simulink model "Dual_Clutch_Trans_SDO_ORIG"  (R2015b)
settings: Solver=ode1  StartTime=0.0  StopTime=15  MaxStep=0.1  RelTol=1e-3
PreLoadFcn:
  | load UrbanCycle1;
  | load UrbanCycle2;
  | load UrbanCycle3;
  | load UrbanCycle4;
  | load UrbanCycle5;
  | load UrbanCycle6;
  | load UrbanCycle7;
  | load UrbanCycle8;
  | Shift_Gear_Delay = 50;
  | Ratio_Time_Const = 0.1;
  | Drive_Cycle_Num = 7;
  | load RefRPMData;
PostLoadFcn:
  | warning off Simulink:SampleTime:TsPropEnabOutputsChangeNotAligned;
  | warning off Simulink:blocks:MatchingFromNotFound
  | warning off Simulink:blocks:MatchingGotoNotFound
  | warning off Simulink:Engine:OutputNotConnected
  | warning off Simulink:Engine:LineWithoutDst
  | warning off Simulink:Engine:UINotUpdatedDuringRapidAccelSim
  | warning off Simulink:Commands:SetParamLinkChangeWarn
  | warning off Simulink:Engine:SaveWithParameterizedLinks_Warning
undefined symbols (not defined in the file or in its folder): DCT_Param, Downshift_Speeds, sigbuilder_block, Upshift_Speeds
libraries: fl_lib x8, nesl_utility x7, sdl_lib x3, simulink x3, DCT_Vehicle_Dynamics_Lib x1
(part 1 of 2)
Description:
  | Vehicle With Dual Clutch Transmission
  | 
  | The vehicle simulated in this demo has a five-speed automatic dual-clutch
  | transmission. The transmission controller converts the pedal deflection
  | into a demanded torque. This demanded torque is then passed to the
  | engine management. The pedal deflection and the vehicle speed are also
  | used by the transmission controller to determine when the gear shifts
  | should occur. Gear shifts are implemented via the two clutches, one clutch
  | pressure being ramped up as the other clutch pressure is ramped down.
  | Gear pre-selection is used to ensure that the correct gear is fully selected
  | before the on-going clutch is enabled. Double-click on the two blocks
  | labeled "Configure for ...." to switch between variable and fixed-step solvers.
  | 
  | 
  | Copyright 2008-2016 The MathWorks, Inc.
settings Model: ParamWorkspaceSource=ReferencedWorkspace  ExtModeTrigDuration=200  ExtModeLogAll=off  TunableVars=Downshift_Speeds,Pedal_Positions,Upshift_Speeds  TunableVarsStorageClass=Auto,Auto,Auto  TunableVarsTypeQualifier=,,  Creator=MathWorks  LastModifiedBy=smiller
settings SolverCC: MaxConsecutiveZCs=10  MaxConsecutiveMinStep=5  EnableConcurrentExecution=on  AutoInsertRateTranBlk=on
settings DataIOCC: MaxDataPoints=1  SaveFormat=StructureWithTime  SaveOutput=off  DSMLogging=off  SaveTime=off  SignalLoggingName=SDO_logsout
settings OptimizationCC: BlockReduction=off  DefaultParameterBehavior=Inlined  OptimizeBlockIOStorage=off  BufferReuse=off  GlobalBufferReuse=off  ExpressionFolding=off  ExpressionDepthLimit=2147483647  LocalBlockOutputs=off
settings DebuggingCC: AlgebraicLoopMsg=error  UnderspecifiedInitializationDetection=Classic  MergeDetectMultiDrivingBlocksExec=none  IgnoredZcDiagnostic=none  MultiTaskRateTransMsg=warning  FcnCallInpInsideContextMsg=UseLocalSettings  StateNameClashWarn=warning
settings HardwareCC: ProdBitPerPointer=32  ProdLargestAtomicFloat=None  ProdWordSize=32  ProdLongLongMode=on  ProdHWDeviceType=Generic->32-bit x86 compatible
settings RTWCC: SystemTargetFile=slrt.tlc  TemplateMakefile=slrt_default_tmf  Description=Simulink Real-Time  RTWCompilerOptimization=on
settings ConfigComp: CovModelRefEnable=Off
settings SimscapeCC: ExplicitSolverDiagnosticOptions=none  SimscapeLogLimitData=off  SimscapeLogDataHistory=50000

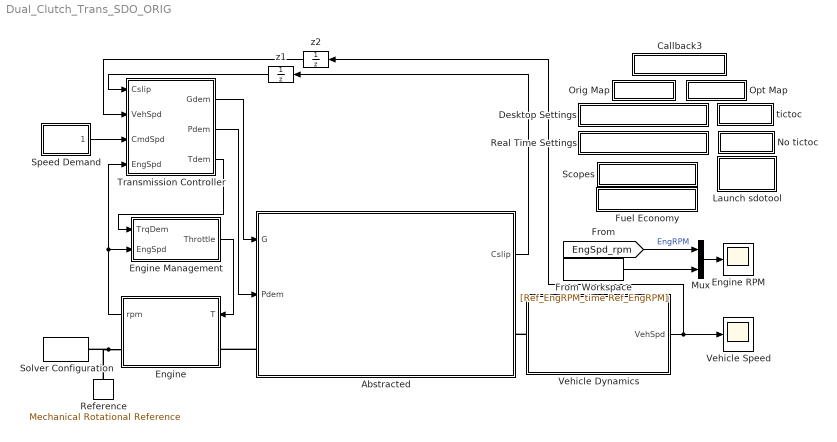
== system Dual_Clutch_Trans_SDO_ORIG ==
  Abstracted : Subsystem
      mask Display:
      | image(imread('DCT_Transmission_Abstracted_IMAGE2.jpg'));
      | port_label('input',1,'G')
      | port_label('input',2,'Pdem')
      | port_label('output',1,'Cslip')
      | color('red');
      | port_label('LConn',1,'B')
      | port_label('RConn',1,'F')
  Callback3 : Subsystem
      settings: OpenFcn=Plot_Gear_Shift_Schedule(Pedal_Positions,Upshift_Speeds, Downshift_Speeds);
      mask Display: disp('Shift Schedule')
  Desktop Settings : Subsystem
      settings: OpenFcn=|
      | set_param(gcs,'solver','ode23t')
      | set_param(sprintf([gcs '/Solver\nConfiguration']),'UseLocalSolver','off')
      | 
      | set_param(sprintf([gcs '/Solver\nConfiguration']),'DoFixedCost','off')
      mask Display: disp('Desktop Settings')
  Engine : Subsystem
      mask Display:
      | plot([200.294537656123;201.704177092068;202.879954177142;203.81054553527;204.486989062962;204.902770239264;205.053884864158;204.938877621199;204.558856093007;203.917480094638;203.02092642757;201.877829393721;200.499197642409;198.898308151034;197.090578360535;195.093417696999;192.926059909376;191.349221415216], [79.0962651705123;81.4129472419303;83.856642682368;86.4038173688741;89.0299406167901;91.7097214236537;94.4173520353776;97.1267564890293;99.8118417386092;102.446748945347;105.006102512455;107.465254465996;109.80052182835;111.989414698229;114.010852840726;115.845368701499;117.475294889959;118.468271604945])
      | plot([180.070315486255;177.215173525063;174.340173090774;171.473002009205;168.641272705228;165.872256280019;163.192619875453;160.628169854943;158.203603274058;155.942270034374;153.865948011161;151.994633320535;150.346347745932;148.936965178479;147.780058742747;146.886770080143;146.265702048809;145.922835873396;145.861473542603;146.08220600922;146.58290749893;147.358755982674;148.402279615432;149.703428694174;151.249672441989;153.026119686324;155.015662269112;157.199139807684;159.555524219735;162.062122235246;164.694793945081;167.42818528151;170.23597219174;173.091114152932;175.966114587221;178.83328566879;181.665014972767;184.434031397976;185.486929355725], [123.25590763568;123.598773811093;123.660136141886;123.439403675268;122.938702185559;122.162853701815;121.119330069056;119.818180990315;118.2719372425;116.495489998164;114.505947415377;112.322469876805;109.966085464754;107.459487449243;104.826815739408;102.093424402979;99.2856374927491;96.4304955315569;93.5554950972677;90.688324015699;87.8565947117214;85.0875782865128;82.4079418819464;79.8434918614364;77.4189252805513;75.1575920408679;73.081270017655;71.2099553270291;69.5616697524256;68.1522871849724;66.9953807492411;66.1020920866371;65.4810240553025;65.1381578798894;65.0767955490969;65.2975280157144;65.7982295054238;66.5740779891678;66.9481130562871])
      | plot([182.088349247351;182.056804583223;181.962474383197;181.806267098667;181.589687091173;181.314820144583;180.98431337785;180.601349751811;180.169617415534;179.693274187426;179.176907513169;178.625490286111;178.044332955585;177.439032384376;176.815417947876;176.17949539401;175.537389004603;174.895282615196;174.25936006133;173.63574562483;173.030445053621;172.449287723095;171.897870496037;171.38150382178;170.905160593672;170.473428257395;170.090464631356;169.759957864623;169.485090918033;169.268510910539;169.112303626009;169.017973425983;168.986428761855;169.017973425983;169.112303626009;169.268510910539;169.485090918033;169.759957864623;170.090464631356;170.473428257395;170.905160593672;171.38150382178;171.897870496037;172.449287723095;173.030445053621;173.63574562483;174.25936006133;174.895282615196;175.537389004603;176.17949539401;176.815417947876;177.439032384376;178.044332955585;178.625490286111;179.176907513169;179.693274187426;180.169617415534;180.601349751811;180.98431337785;181.314820144583;181.589687091173;181.806267098667;181.962474383197;182.056804583223;182.088349247351;182.088349247351], [94.3432759959251;93.7073437064164;93.0775357924916;92.4599176486499;91.8604372752408;91.2848679959696;90.7387528576339;90.2273512475527;89.7555882427917;89.3280071789786;88.9487258954975;88.6213970784445;88.3491730832641;88.1346755758426;87.9799702844327;87.8865471055612;87.8553057555109;87.8865471055612;87.9799702844327;88.1346755758426;88.3491730832641;88.6213970784445;88.9487258954975;89.3280071789786;89.7555882427917;90.2273512475527;90.7387528576339;91.2848679959696;91.8604372752408;92.4599176486499;93.0775357924916;93.7073437064164;94.3432759959251;94.9792082854337;95.6090161993586;96.2266343432003;96.8261147166093;97.4016839958805;97.9477991342162;98.4592007442974;98.9309637490584;99.3585448128716;99.7378260963527;100.065154913406;100.337378908586;100.551876416008;100.706581707417;100.800004886289;100.831246236339;100.800004886289;100.706581707417;100.551876416008;100.337378908586;100.065154913406;99.7378260963526;99.3585448128716;98.9309637490584;98.4592007442974;97.9477991342162;97.4016839958805;96.8261147166093;96.2266343432003;95.6090161993586;94.9792082854338;94.3432759959251;94.3432759959251])
      | plot([201.615249970928;201.583705306799;201.489375106774;201.333167822243;201.11658781475;200.84172086816;200.511214101427;200.128250475388;199.69651813911;199.220174911002;198.703808236745;198.152391009688;197.571233679162;196.965933107953;196.342318671452;195.706396117586;195.06428972818;194.422183338773;193.786260784907;193.162646348407;192.557345777197;191.976188446671;191.424771219614;190.908404545357;190.432061317249;190.000328980971;189.617365354932;189.286858588199;189.011991641609;188.795411634116;188.639204349585;188.54487414956;188.513329485431;188.54487414956;188.639204349585;188.795411634116;189.011991641609;189.286858588199;189.617365354932;190.000328980971;190.432061317249;190.908404545357;191.424771219614;191.976188446671;192.557345777197;193.162646348407;193.786260784907;194.422183338773;195.06428972818;195.706396117586;196.342318671452;196.965933107953;197.571233679162;198.152391009688;198.703808236745;199.220174911002;199.69651813911;200.128250475388;200.511214101427;200.84172086816;201.11658781475;201.333167822243;201.489375106774;201.583705306799;201.615249970928;201.615249970928], [74.7533852700144;74.1174529805057;73.487645066581;72.8700269227392;72.2705465493302;71.694977270059;71.1488621317233;70.6374605216421;70.165697516881;69.7381164530679;69.3588351695868;69.0315063525339;68.7592823573535;68.5447848499319;68.390079558522;68.2966563796505;68.2654150296003;68.2966563796505;68.390079558522;68.5447848499319;68.7592823573535;69.0315063525339;69.3588351695868;69.7381164530679;70.165697516881;70.6374605216421;71.1488621317233;71.694977270059;72.2705465493302;72.8700269227392;73.487645066581;74.1174529805057;74.7533852700144;75.3893175595231;76.0191254734479;76.6367436172896;77.2362239906986;77.8117932699698;78.3579084083055;78.8693100183867;79.3410730231478;79.7686540869609;80.147935370442;80.4752641874949;80.7474881826754;80.9619856900969;81.1166909815068;81.2101141603783;81.2413555104285;81.2101141603783;81.1166909815068;80.9619856900969;80.7474881826753;80.4752641874949;80.147935370442;79.7686540869609;79.3410730231478;78.8693100183867;78.3579084083055;77.8117932699698;77.2362239906986;76.6367436172896;76.0191254734479;75.3893175595231;74.7533852700145;74.7533852700144])
      | plot([201.615249970928;201.583705306799;201.489375106774;201.333167822243;201.11658781475;200.84172086816;200.511214101427;200.128250475388;199.69651813911;199.220174911002;198.703808236745;198.152391009688;197.571233679162;196.965933107953;196.342318671452;195.706396117586;195.06428972818;194.422183338773;193.786260784907;193.162646348407;192.557345777197;191.976188446671;191.424771219614;190.908404545357;190.432061317249;190.000328980971;189.617365354932;189.286858588199;189.011991641609;188.795411634116;188.639204349585;188.54487414956;188.513329485431;188.54487414956;188.639204349585;188.795411634116;189.011991641609;189.286858588199;189.617365354932;190.000328980971;190.432061317249;190.908404545357;191.424771219614;191.976188446671;192.557345777197;193.162646348407;193.786260784907;194.422183338773;195.06428972818;195.706396117586;196.342318671452;196.965933107953;197.571233679162;198.152391009688;198.703808236745;199.220174911002;199.69651813911;200.128250475388;200.511214101427;200.84172086816;201.11658781475;201.333167822243;201.489375106774;201.583705306799;201.615249970928;201.615249970928], [74.7533852700144;74.1174529805057;73.487645066581;72.8700269227392;72.2705465493302;71.694977270059;71.1488621317233;70.6374605216421;70.165697516881;69.7381164530679;69.3588351695868;69.0315063525339;68.7592823573535;68.5447848499319;68.390079558522;68.2966563796505;68.2654150296003;68.2966563796505;68.390079558522;68.5447848499319;68.7592823573535;69.0315063525339;69.3588351695868;69.7381164530679;70.165697516881;70.6374605216421;71.1488621317233;71.694977270059;72.2705465493302;72.8700269227392;73.487645066581;74.1174529805057;74.7533852700144;75.3893175595231;76.0191254734479;76.6367436172896;77.2362239906986;77.8117932699698;78.3579084083055;78.8693100183867;79.3410730231478;79.7686540869609;80.147935370442;80.4752641874949;80.7474881826754;80.9619856900969;81.1166909815068;81.2101141603783;81.2413555104285;81.2101141603783;81.1166909815068;80.9619856900969;80.7474881826753;80.4752641874949;80.147935370442;79.7686540869609;79.3410730231478;78.8693100183867;78.3579084083055;77.8117932699698;77.2362239906986;76.6367436172896;76.0191254734479;75.3893175595231;74.7533852700145;74.7533852700144])
      | plot([142.90856779553;142.90856779553;208.103220211342;208.103220211342], [139.948037685826;218.181620584801;218.181620584801;139.948037685826])
      | plot([142.90856779553;208.103220211342], [179.064829135314;179.064829135314])
      | plot([149.459528038278;149.459528038278], [179.064829135314;172.576858894899])
      | plot([201.615249970928;201.615249970928], [179.064829135314;172.576858894899])
      | plot([142.90856779553;208.103220211342;208.103220211342;142.90856779553;142.90856779553], [179.064829135314;179.064829135314;152.986968168989;152.986968168989;179.064829135314])
      | plot([142.90856779553;208.103220211342], [192.103759618476;192.103759618476])
      | plot([180.639579193667;200.229469919577], [99.0045361686498;79.4776354450732])
      | plot([173.332738922909;192.92262964882], [87.8553057555109;68.3284050319344])
      | plot([183.663099305704;200.481429928914], [153.553878189996;76.9580353517085])
      | plot([184.544959338382;174.970478983596], [95.0361660216004;153.553878189996])
      | plot([183.474129298702;186.749609420076;206.654450157657;201.615249970928;197.961829835549], [76.9580353517085;62.0923948008567;67.8874750155956;88.1702557671815;87.7923157531768])
      | plot([164.199188584462;187.694459455088], [94.7842060122639;95.1621460262686])
      | plot([175.537389004603;175.285428995267], [106.50034644641;81.9342455361038])
      | plot([142.90856779553;208.103220211342], [172.576858894899;172.576858894899])
      | plot([297.86397353746;357.389525743201], [71.0999651346356;71.0999651346356])
      | plot([269.518472487107;297.86397353746;297.86397353746;269.518472487107;269.518472487107], [85.2727156598121;85.2727156598121;56.927214609459;56.927214609459;85.2727156598121])
      | plot([258.180272066966;269.518472487107;269.518472487107;258.180272066966], [42.7544640842825;42.7544640842825;99.4454661849886;99.4454661849886])
      | plot([108.893966535106;108.245686045801;107.603648851995;106.974038122836;106.362917353826;105.776171972045;105.219452656266;104.698120917834;104.217197466378;103.781313857637;103.394667889039;103.060983172626;102.783473274627;102.564810767061;102.40710148941;102.31186426823;102.280016290024;102.280016290024;102.31186426823;102.40710148941;102.564810767061;102.783473274627;103.060983172626;103.394667889039;103.781313857637;104.217197466378;104.698120917834;105.219452656266;105.776171972045;106.362917353826;106.974038122836;107.603648851995;108.245686045801;108.893966535106;249.67662175186;250.324902241165;250.966939434972;251.596550164131;252.20767093314;252.794416314921;253.3511356307;253.872467369133;254.353390820588;254.78927442933;255.175920397927;255.50960511434;255.787115012339;256.005777519905;256.163486797556;256.258724018736;256.290571996942;256.290571996942;256.258724018736;256.163486797556;256.005777519905;255.787115012339;255.50960511434;255.175920397927;254.78927442933;254.353390820588;253.872467369133;253.3511356307;252.794416314921;252.20767093314;251.596550164131;250.966939434972;250.324902241165;249.67662175186;108.893966535106], [233.173241140321;233.141393162114;233.046155940935;232.888446663284;232.669784155718;232.392274257719;232.058589541306;231.671943572708;231.236059963967;230.755136512511;230.233804774079;229.6770854583;229.090340076519;228.479219307509;227.84960857835;227.207571384544;226.559290895239;46.5338642243296;45.8855837350246;45.2435465412178;44.6139358120588;44.0028150430496;43.4160696612682;42.8593503454891;42.3380186070568;41.8570951556014;41.4212115468599;41.0345655782626;40.7008808618494;40.42337096385;40.2047084562844;40.0469991786335;39.9517619574538;39.9199139792472;39.9199139792472;39.9517619574538;40.0469991786335;40.2047084562844;40.42337096385;40.7008808618494;41.0345655782626;41.4212115468599;41.8570951556014;42.3380186070568;42.8593503454891;43.4160696612682;44.0028150430496;44.6139358120588;45.2435465412178;45.8855837350246;46.5338642243296;226.559290895239;227.207571384544;227.84960857835;228.479219307509;229.090340076519;229.6770854583;230.233804774079;230.755136512511;231.236059963967;231.671943572708;232.058589541306;232.392274257719;232.669784155718;232.888446663284;233.046155940935;233.141393162114;233.173241140321;233.173241140321])
      | patch([0;354.791188146919;354.791188146919;0;0;0.472425017505884;0.472425017505884;354.318763129413;354.318763129413;0.472425017505884;0], [283.927435521036;283.927435521036;0;0;283.927435521036;283.455010503531;0.472425017505884;0.472425017505884;283.455010503531;283.455010503531;283.927435521036], [1;1;1])
      | plot([102.280016290024;0.236212508752942], [71.0999651346356;71.0999651346356])
      | ;
      | color('black');
      | port_label('input', 1,'T')
      | port_label('output', 1,'rpm')
      | port_label('RConn', 1,'B')
      | port_label('LConn', 1,'F')
  Engine Management : Subsystem
  Engine RPM : Scope
  From Workspace : FromWorkspace  VariableName=[Ref_EngRPM_time Ref_EngRPM]  SampleTime=0.01
  Fuel Economy : Subsystem  mask(Data Acquisition){}
      mask Display: disp('Fuel Economy');
  Launch sdotool : Subsystem
      settings: OpenFcn=|
      | load([bdroot '_sdosession']);
      | sdotool(SDOSessionData);
      mask Display: disp('Launch\nsdotool')
  Mux : Mux  Inputs=2
  No tictoc : Subsystem
      settings: OpenFcn=|
      | set_param(bdroot,'StartFcn','');
      | set_param(bdroot,'StopFcn','');
      mask Display: disp('No tictoc')
  Opt Map : Subsystem
      settings: OpenFcn=|
      | Upshift_Speeds = DCT_Param.Shift_Map_OPT.Upshift_Speeds;
      | Downshift_Speeds = DCT_Param.Shift_Map_OPT.Downshift_Speeds;
      | Pedal_Positions = DCT_Param.Shift_Map_OPT.Pedal_Positions;
      mask Display: disp('Opt Map')
  Orig Map : Subsystem
      settings: OpenFcn=|
      | Upshift_Speeds = DCT_Param.Shift_Map_ORIG.Upshift_Speeds;
      | Downshift_Speeds = DCT_Param.Shift_Map_ORIG.Downshift_Speeds;
      | Pedal_Positions = DCT_Param.Shift_Map_ORIG.Pedal_Positions;
      mask Display: disp('Orig Map')
  Real Time Settings : Subsystem
      settings: OpenFcn=|
      | set_param(gcs,'solver','ode1')
      | set_param(sprintf([gcs '/Solver\nConfiguration']),'UseLocalSolver','on')
      | 
      | set_param(sprintf([gcs '/Solver\nConfiguration']),'DoFixedCost','on')
      mask Display: disp('Real Time Settings')
  Reference : fl_lib/Mechanical/Rotational Elements/Mechanical Rotational Reference
  Scopes : Subsystem
      mask Display: disp('Scopes')
  Solver Configuration : nesl_utility/Solver Configuration  PhysicalDomain=network_engine_domain  SubClassName=solver  LeftPortType=input  RightPortType=generic  Accelerate=off  Tones=[]  Harmonics=[]  SimulateNoise=off  Profile=off  UseLocalSampling=off  EnableSwitchedLinearOptims=on  FrequencyDomain=off  UseCCode=off  RelTol=0.001  AbsTol=1e-06  MinStep=1e-09  ToWorkspace=off  RevertToSquareIcSolve=off  NumHomotopyIterations=100  PhasorMode=off  PhasorModeNumHarmonics=1  DoDC=off  ResidualTolerance=1e-9  UseLocalSolver=on  LocalSolverChoice=NE_BACKWARD_EULER_ADVANCER  LocalSolverSampleTime=.005  DoFixedCost=on  MaxNonlinIter=2  MaxModeIter=2  LinearAlgebra=Sparse  DelaysMemoryBudget=1024  AutomaticFiltering=on  FilteringTimeConstant=0.001
  Speed Demand : Subsystem
      mask Display:
      | plotstr=['UrbanCycle' evalin('base','num2str(Drive_Cycle_Num)')];
      | plot(evalin('base',[plotstr '.time']),evalin('base',[plotstr '.SpdKph']));
      | text(evalin('base',['0.7*max(' plotstr '.time)']),evalin('base',['0.25*max(' plotstr '.SpdKph)']),evalin('base','num2str(Drive_Cycle_Num)'));
  Transmission Controller : Subsystem
  Vehicle Dynamics : Subsystem  BlockChoice=Simple
      settings: AttributesFormatString=%<BlockChoice>  TemplateBlock=DCT_Vehicle_Dynamics_Lib/Vehicle Dynamics  MemberBlocks=Full,Simple
      mask Display:
      | port_label('LConn',1,'Sh');
      | port_label('output',1,'Spd');
  Vehicle Speed : Scope
  tictoc : Subsystem
      settings: OpenFcn=|
      | set_param(bdroot,'StartFcn','tic;');
      | set_param(bdroot,'StopFcn','Elapsed_Sim_Time = toc; disp([''Elapsed time for '' bdroot '' = '' num2str(Elapsed_Sim_Time)])');
      mask Display: disp('tictoc')
  z1 : UnitDelay  SampleTime=0.01
  z2 : UnitDelay  SampleTime=0.01
  wires:
  Transmission Controller/2(Pdem) -> Abstracted/2(Pdem)
  Transmission Controller/1(Gdem) -> Abstracted/1(G)
  z1/1 -> Transmission Controller/1(Cslip)
  Engine Management/1(Throttle) -> Engine/1(T)
  Transmission Controller/3(Tdem) -> Engine Management/1(TrqDem)
  Engine/1(rpm) -> Transmission Controller/4(EngSpd), Engine Management/2(EngSpd)
  Abstracted/1(Cslip) -> z1/1
  Vehicle Dynamics/1(VehSpd) -> Vehicle Speed/1, z2/1
  Speed Demand/1(Speed Command) -> Transmission Controller/3(CmdSpd)
  z2/1 -> Transmission Controller/2(VehSpd)
  [EngSpd_rpm] -> Mux/1  "EngRPM"
  From Workspace/1 -> Mux/2
  Mux/1 -> Engine RPM/1
  connections:
  Engine/RConn1 -- Reference/LConn1 -- Solver Configuration/RConn1
  Abstracted/LConn1 -- Engine/LConn1
  Vehicle Dynamics/LConn1 -- Abstracted/RConn1

== system Dual_Clutch_Trans_SDO_ORIG/Abstracted ==
  G : Inport
  Pdem : Inport  Port=2
  Clutches : Subsystem
      mask Display: image(imread('DCT_Clutches_Abstracted_IMAGE.jpg'));
  Gears : Subsystem
      mask Display: image(imread('DCT_Gears_Abstracted_IMAGE.jpg'));
  Shaft Inertia Output Shaft : fl_lib/Mechanical/Rotational Elements/Inertia  inertia=DCT_Param.Transmission.Shaft_Inertia_Output kg*m^2  w_specify=on  w_priority=High  w=DCT_Param.Transmission.Shaft_Velocity_Output rad/s  t_specify=off  t_priority=None  t=0 N*m
  B : PMIOPort  Port=1  Side=Left
  F : PMIOPort  Port=2  Side=Right
  Cslip : Outport
  wires:
  Pdem/1 -> Clutches/1(Pdem)
  Clutches/1(Cslip) -> Cslip/1
  G/1 -> Gears/1(G)
  connections:
  B/RConn1 -- Clutches/LConn1
  Clutches/RConn1 -- Gears/LConn1
  Gears/RConn1 -- F/RConn1 -- Shaft Inertia Output Shaft/LConn1

== system Dual_Clutch_Trans_SDO_ORIG/Callback3 ==

== system Dual_Clutch_Trans_SDO_ORIG/Desktop Settings ==

== system Dual_Clutch_Trans_SDO_ORIG/Engine ==
  T : Inport
  Generic Engine : sdl_lib/Engines/Generic Engine  model_parameterization=1  engine_type=1  P_max=DCT_Param.ICE.Max_Power W  w_P_max=DCT_Param.ICE.Speed_At_Max_Power rpm  w_max=DCT_Param.ICE.Max_Speed rpm  w_min=DCT_Param.ICE.Stall_Speed rpm  w_tab=[ 500 1000 2e+3 3e+3 4e+3 5e+3 6e+3 7e+3 ] rpm  trq_tab=[ 380 380 380 380 350 280 200 80 ] N*m  pwr_tab=[ 2e+4 4e+4 7.8e+4 1.2e+5 1.45e+5 1.48e+5 1.25e+5 6e+4 ] W  interp_method=1  model_inertia=1  inertia=DCT_Param.ICE.Shaft_Inertia kg*m^2  initial_velocity=DCT_Param.ICE.Initial_Velocity rpm  model_time_constant=1  time_constant=DCT_Param.ICE.Engine_Time_Constant s  T0=DCT_Param.ICE.Initial_Normalized_Throttle  w_thr=DCT_Param.ICE.Speed_Threshold rpm  idle_speed=0  idle_speed_reference=1000 rpm  tau_controller=1 s  idle_w_thr=1 rpm  fc_model=1  fc_per_rev=25 mg/rev  displaced_volume=400 cm^3  rev_per_cycle=2  fc_w_tab=[ 1000 2e+3 3e+3 4e+3 5e+3 6e+3 ] rpm  fc_trq_tab=[ 0 80 160 200 240 320 360 400 ] N*m  fc_tab=[ 0.5 0.9 1.4 1.6 1.9 2.7 3.4 4.4; 1 1.7 2.7 3.1 3.6 5 6 7.4; 1.4 2.7 4 4.8 5.6 7.5 8.5 10.5; 2 3.6 5.8 6.7 8 10.4 11.7 13.3; 2.5 4.8 7.9 9.4 10.8 14 16.2 18.6; 3.1 6 10.3 11.9 13.8 18.4 22 26.5 ] g/s  bmep_tab=[ 0 250 500 625 750 1000 1.15e+3 1.25e+3 ] kPa  bsfc_tab=[ 410 380 300 280 270 290 320 380; 410 370 290 270 260 270 285 320; 415 380 290 275 265 270 270 300; 420 390 310 290 285 280 280 285; 430 410 340 320 310 300 310 320; 450 430 370 340 330 330 350 380 ] g/hr/kW  fc_interp_method=1
  Rate Transition : RateTransition
  Simulink-PS Converter : nesl_utility/Simulink-PS Converter  PhysicalDomain=network_engine_domain  SubClassName=ps_input  LeftPortType=input  RightPortType=output  PseudoPeriodic=off  Frequencies=[]  NoiseDistribution=none  NoiseParameters=[]  Unit=1  AffineConversion=off  InputFiltering=off  SimscapeFilterOrder=1  InputFilterTimeConstant=.001  UdotUserProvided=0
  Torque Sensor : Subsystem
      mask Display: disp('S')
  Velocity sensor : Subsystem
      mask Display: disp('S')
  F : PMIOPort  Port=1  Side=Left
  B : PMIOPort  Port=2  Side=Right
  rpm : Outport
  wires:
  T/1 -> Rate Transition/1
  Velocity sensor/1(rpm) -> rpm/1
  Rate Transition/1 -> Simulink-PS Converter/1
  connections:
  Simulink-PS Converter/RConn1 -- Generic Engine/LConn1
  B/RConn1 -- Generic Engine/LConn2
  Torque Sensor/RConn1 -- F/RConn1
  Velocity sensor/LConn1 -- Generic Engine/RConn3 -- Torque Sensor/LConn1

== system Dual_Clutch_Trans_SDO_ORIG/Engine Management ==
  TrqDem : Inport
  EngSpd : Inport  Port=2
  Constant : Constant  Value=0  SampleTime=0.01
  Idle rpm reference demand : Constant  Value=DCT_Param.ICE.Idle_Ref_Spd  SampleTime=0.01
  Inhibit idle speed controller if THdem>0.02 : Switch  Threshold=0.02  InputSameDT=on
  Inverse engine map : Subsystem  mask(Inverse engine map){P0=92000, rpm0=5500}
      mask prompts: P0 "Engine maximum power (W)"; rpm0 "Speed at maximum power (rpm)"
      mask help: Converts measured speed and demanded torque into normalized throttle demand. Assumes that the engine is modeled using the SimDriveline Generic Engine block with model parameterization set to Normalized 3rd-order polynomial matched to peak power.
      mask init:
      | w0 = 2*pi*rpm0/60;
  Kp : Gain  Gain=0.005*2*pi/60  SaturateOnIntegerOverflow=on  OutDataTypeStr=Inherit: Same as input  ParamDataTypeStr=Inherit: Same as input
  Sum1 : Sum  Inputs=++|  SaturateOnIntegerOverflow=on  InputSameDT=on  OutDataTypeStr=Inherit: Same as first input
  Sum2 : Sum  Inputs=+-|  SaturateOnIntegerOverflow=on  InputSameDT=on  OutDataTypeStr=Inherit: Same as first input
  "[-0.02,0.02]" : Saturate  UpperLimit=0.02  LowerLimit=-0.02
  Throttle : Outport
  tag scope: throttle=global
  wires:
  Inverse engine map/1(throttle) -> [throttle], Sum1/2, Inhibit idle speed controller if THdem>0.02/2  "THdem"
  TrqDem/1 -> Inverse engine map/2(trq_demand)
  EngSpd/1 -> Inverse engine map/1(EngSpd), Sum2/2
  Inhibit idle speed controller if THdem>0.02/1 -> Sum1/1
  Constant/1 -> Inhibit idle speed controller if THdem>0.02/3
  Sum1/1 -> Throttle/1
  Idle rpm reference demand/1 -> Sum2/1
  Sum2/1 -> Kp/1
  Kp/1 -> "[-0.02,0.02]"/1
  "[-0.02,0.02]"/1 -> Inhibit idle speed controller if THdem>0.02/1

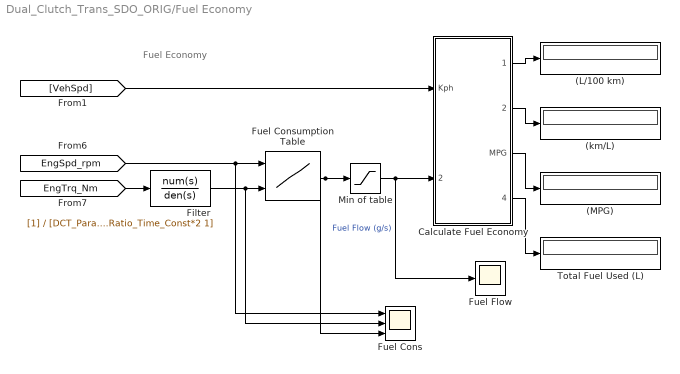
== system Dual_Clutch_Trans_SDO_ORIG/Fuel Economy ==
  note: Fuel Economy
  (L/100 km) : Display
      settings: Decimation=decimation
  (MPG) : Display
      settings: Decimation=decimation
  (km/L) : Display
      settings: Decimation=decimation
  Calculate Fuel Economy : Subsystem
  Filter : TransferFcn  Denominator=[DCT_Param.Transmission.Abstract.Ratio_Time_Const*2 1]
  Fuel Consumption Table : Lookup2D  RowIndex=DCT_Param.ICE.FC.Speed_Vector  ColumnIndex=DCT_Param.ICE.FC.Torque_Vector  Table=DCT_Param.ICE.FC.Consumption_Table
  Fuel Cons : Scope  NumInputPorts=3
  Fuel Flow : Scope
  Min of table : Saturate  UpperLimit=Inf  LowerLimit=min(min(DCT_Param.ICE.FC.Consumption_Table))
  Total Fuel Used (L) : Display
      settings: Decimation=decimation
  wires:
  Calculate Fuel Economy/1(Liter/100Km) -> (L/100 km)/1
  Calculate Fuel Economy/3(MPG) -> (MPG)/1
  [VehSpd] -> Calculate Fuel Economy/1(Kph)
  Calculate Fuel Economy/4(Fuel Used (L)) -> Total Fuel Used (L)/1
  Calculate Fuel Economy/2(Km/Liter) -> (km/L)/1
  Fuel Consumption Table/1 -> Fuel Cons/3, Min of table/1
  [EngSpd_rpm] -> Fuel Consumption Table/1, Fuel Cons/1
  [EngTrq_Nm] -> Filter/1
  Filter/1 -> Fuel Consumption Table/2, Fuel Cons/2
  Min of table/1 -> Calculate Fuel Economy/2(Fuel Flow g/s), Fuel Flow/1  "Fuel Flow (g/s)"

== system Dual_Clutch_Trans_SDO_ORIG/Launch sdotool ==

== system Dual_Clutch_Trans_SDO_ORIG/No tictoc ==

== system Dual_Clutch_Trans_SDO_ORIG/Opt Map ==

== system Dual_Clutch_Trans_SDO_ORIG/Orig Map ==

== system Dual_Clutch_Trans_SDO_ORIG/Real Time Settings ==

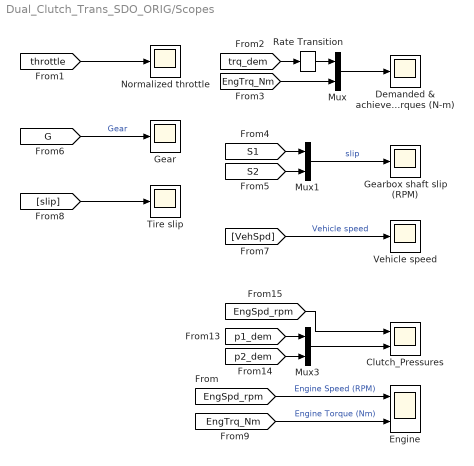
== system Dual_Clutch_Trans_SDO_ORIG/Scopes ==
  Clutch_Pressures : Scope  NumInputPorts=2
  Demanded & achieved torques (N-m) : Scope
  Engine : Scope  NumInputPorts=2
  Gear : Scope
  Gearbox shaft slip (RPM) : Scope
  Mux : Mux  Inputs=2
  Mux1 : Mux  Inputs=2
  Mux3 : Mux  Inputs=2
  Normalized throttle : Scope
  Rate Transition : RateTransition
  Tire slip : Scope
  Vehicle speed : Scope
  wires:
  [throttle] -> Normalized throttle/1
  Mux/1 -> Demanded & achieved torques (N-m)/1
  [EngTrq_Nm] -> Mux/2
  Mux1/1 -> Gearbox shaft slip (RPM)/1  "slip"
  [S1] -> Mux1/1
  [S2] -> Mux1/2
  [G] -> Gear/1  "Gear"
  [VehSpd] -> Vehicle speed/1  "Vehicle speed"
  [slip] -> Tire slip/1
  Mux3/1 -> Clutch_Pressures/2
  [p1_dem] -> Mux3/1
  [p2_dem] -> Mux3/2
  [EngSpd_rpm] -> Clutch_Pressures/1
  [trq_dem] -> Rate Transition/1
  Rate Transition/1 -> Mux/1
  [EngSpd_rpm] -> Engine/1  "Engine Speed (RPM)"
  [EngTrq_Nm] -> Engine/2  "Engine Torque (Nm)"

== system Dual_Clutch_Trans_SDO_ORIG/Speed Demand ==
  "10-15 mode " : Subsystem  Tag=STV Subsys  LoadFcn=sigbuilder_block('load');  StartFcn=sigbuilder_block('start');  StopFcn=sigbuilder_block('stop');  ClipboardFcn=sigbuilder_block('clipboard');  mask(Sigbuilder block){}
      mask help: Sigbuilder GUI
      mask init:
      | if ~strcmp(get_param(bdroot(gcbh),'SimulationStatus'),'stopped') tuvar = sigbuilder_block('maskInit'); end
      settings: CopyFcn=sigbuilder_block('copy');  DeleteFcn=sigbuilder_block('delete');  ModelCloseFcn=sigbuilder_block('modelClose');  PreSaveFcn=sigbuilder_block('preSave');  PauseFcn=sigbuilder_block('pause')  ContinueFcn=sigbuilder_block('continue')  NameChangeFcn=sigbuilder_block('namechange');  OpenFcn=sigbuilder_block('open',[561.75 178.5 550.5 399 ]);  CloseFcn=sigbuilder_block('close');
      mask Display: plot(0,0,100,100,[10,10,40,40,10],[80,20,20,80,80],[40,10],[50,50], [40,27,10],[65,72,56],[40,25,25,10],[28,28,43,43]);
  FTP75 : FromWorkspace  VariableName=[UrbanCycle4.time UrbanCycle4.SpdKph]  SampleTime=0
  FTP75 Transient : FromWorkspace  VariableName=[UrbanCycle8.time UrbanCycle8.SpdKph]  SampleTime=0
  FTP75 short : FromWorkspace  VariableName=[UrbanCycle7.time UrbanCycle7.SpdKph]  SampleTime=0
  Multiport Switch : MultiPortSwitch  Inputs=8
  Select Cycle : Constant  Value=Drive_Cycle_Num
  Urban Cycle 1 : FromWorkspace  VariableName=[UrbanCycle1.time UrbanCycle1.SpdKph]  SampleTime=0
  Urban Cycle 2 : FromWorkspace  VariableName=[UrbanCycle2.time UrbanCycle2.SpdKph]  SampleTime=0
  Urban Cycle 3 : FromWorkspace  VariableName=[UrbanCycle3.time UrbanCycle3.SpdKph]  SampleTime=0
  Wide Open Throttle : FromWorkspace  VariableName=[UrbanCycle4.time UrbanCycle4.SpdKph]  SampleTime=0
  Speed Command : Outport
  wires:
  Urban Cycle 3/1 -> Multiport Switch/4
  Select Cycle/1 -> Multiport Switch/1
  Urban Cycle 2/1 -> Multiport Switch/3
  Urban Cycle 1/1 -> Multiport Switch/2
  FTP75/1 -> Multiport Switch/5
  "10-15 mode "/1(Target speed) -> Multiport Switch/6
  Multiport Switch/1 -> Speed Command/1
  FTP75 short/1 -> Multiport Switch/8
  Wide Open Throttle/1 -> Multiport Switch/7
  FTP75 Transient/1 -> Multiport Switch/9

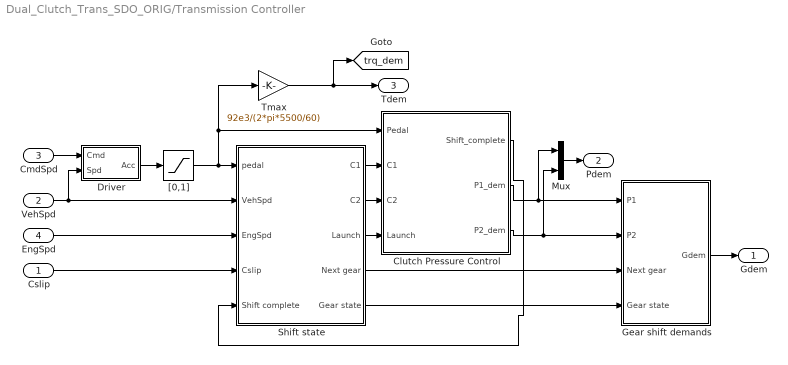
== system Dual_Clutch_Trans_SDO_ORIG/Transmission Controller ==
  Cslip : Inport
  VehSpd : Inport  Port=2
  CmdSpd : Inport  Port=3
  EngSpd : Inport  Port=4
  Clutch Pressure Control : Subsystem
  Driver : Subsystem
  Gear shift demands : Subsystem
  Mux : Mux  Inputs=2
  Shift state : Subsystem
  Tmax : Gain  Gain=92e3/(2*pi*5500/60)  SaturateOnIntegerOverflow=on  OutDataTypeStr=Inherit: Same as input  ParamDataTypeStr=Inherit: Same as input
  "[0,1]" : Saturate  UpperLimit=1  LowerLimit=0
  Gdem : Outport
  Pdem : Outport  Port=2
  Tdem : Outport  Port=3
  tag scope: trq_dem=global
  wires:
  "[0,1]"/1 -> Shift state/1(pedal), Clutch Pressure Control/1(Pedal), Tmax/1
  VehSpd/1 -> Shift state/2(VehSpd), Driver/2(Spd)
  EngSpd/1 -> Shift state/3(EngSpd)
  Cslip/1 -> Shift state/4(Cslip)
  Shift state/5(Gear state) -> Gear shift demands/4(Gear state)
  Shift state/4(Next gear) -> Gear shift demands/3(Next gear)
  Gear shift demands/1(Gdem) -> Gdem/1
  Shift state/1(C1) -> Clutch Pressure Control/2(C1)
  Shift state/2(C2) -> Clutch Pressure Control/3(C2)
  Shift state/3(Launch) -> Clutch Pressure Control/4(Launch)
  Clutch Pressure Control/1(Shift_complete) -> Shift state/5(Shift complete)
  Clutch Pressure Control/3(P2_dem) -> Gear shift demands/2(P2), Mux/2
  Clutch Pressure Control/2(P1_dem) -> Gear shift demands/1(P1), Mux/1
  Tmax/1 -> Tdem/1, [trq_dem]
  Mux/1 -> Pdem/1
  CmdSpd/1 -> Driver/1(Cmd)
  Driver/1(Acc) -> "[0,1]"/1

== system Dual_Clutch_Trans_SDO_ORIG/Vehicle Dynamics ==
  Simple : DCT_Vehicle_Dynamics_Lib/Simple  mass=DCT_Param.Vehicle.Mass  area=DCT_Param.Vehicle.Frontal_Area  Cd=DCT_Param.Vehicle.Aero_Drag_Coeff  radius=DCT_Param.Vehicle.Tire.Radius  wheel_inertia=DCT_Param.Vehicle.Tire.Inertia  gear_ratio=DCT_Param.Vehicle.Final_Drive_Ratio
  Drive Shaft : PMIOPort  Port=1  Side=Left
  VehSpd : Outport
  wires:
  Simple/1 -> VehSpd/1
  connections:
  Simple/LConn1 -- Drive Shaft/RConn1

== system Dual_Clutch_Trans_SDO_ORIG/tictoc ==

== system Dual_Clutch_Trans_SDO_ORIG/Abstracted/Clutches ==
  Pdem : Inport
  Clutch Odd Gears : sdl_lib/Clutches/Disk Friction Clutch  geometry_model=1  r_eff=DCT_Param.Clutch.Torque_Radius mm  d_o=150 mm  d_i=100 mm  nS=DCT_Param.Clutch.Num_Friction_Surfaces  piston_area=DCT_Param.Clutch.Engagement_Piston_Area m^2  unidirectional=0  friction_model=1  mu_coulomb=DCT_Param.Clutch.Kinetic_Friction_Coeff  mu_w_vector=[ 0 0.1 0.2 0.3 0.4 0.5 1 2 5 10 100 1000 ] rad/s  mu_coulomb_vector=[ 0.29 0.28 0.26 0.22 0.21 0.2 0.2 0.19 0.19 0.19 0.19 0.19 ]  mu_interp_method=1  mu_extrap_method=1  mu_static=DCT_Param.Clutch.Static_Friction_Coeff  d_f=DCT_Param.Clutch.Derating_Factor  w_tol=DCT_Param.Clutch.Clutch_Velocity_Tolerance rad/s  pressure_min=DCT_Param.Clutch.Threshold_Pressure Pa  mu_visc=DCT_Param.Clutch.Drag_Torque_Coeff N*m/(rad/s)  initial_state_locked=0
  MinMax : MinMax  Function=max
  Mux : Mux  Inputs=2
  Odd Clutch Actuator : Subsystem
  Shaft Inertia All Gears : fl_lib/Mechanical/Rotational Elements/Inertia  inertia=DCT_Param.Transmission.Shaft_Inertia_Odd kg*m^2  w_specify=on  w_priority=High  w=DCT_Param.Transmission.Shaft_Velocity_Odd rad/s  t_specify=off  t_priority=None  t=0 N*m
  Slip Sensor 2 : Constant  Value=0
  Slip sensor 1 : Subsystem
  Shaft : PMIOPort  Port=1  Side=Right
  E : PMIOPort  Port=2  Side=Left
  Cslip : Outport
  wires:
  Slip sensor 1/1(S1) -> Mux/1
  Mux/1 -> Cslip/1
  Pdem/1 -> MinMax/1
  MinMax/1 -> Odd Clutch Actuator/1(Pdem)
  Slip Sensor 2/1 -> Mux/2
  connections:
  E/RConn1 -- Slip sensor 1/LConn1 -- Clutch Odd Gears/LConn2
  Odd Clutch Actuator/RConn1 -- Clutch Odd Gears/LConn1
  Slip sensor 1/RConn1 -- Clutch Odd Gears/RConn1 -- Shaft/RConn1 -- Shaft Inertia All Gears/LConn1

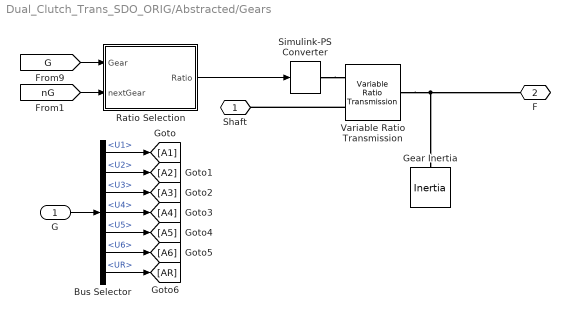
== system Dual_Clutch_Trans_SDO_ORIG/Abstracted/Gears ==
  G : Inport
  Bus Selector : BusSelector  OutputSignals=U1,U2,U3,U4,U5,U6,UR
  Gear Inertia : fl_lib/Mechanical/Rotational Elements/Inertia  inertia=DCT_Param.Transmission.Gear_Inertia kg*m^2  w_specify=on  w_priority=High  w=0 rad/s  t_specify=off  t_priority=None  t=0 N*m
  Ratio Selection : Subsystem
  Simulink-PS Converter : nesl_utility/Simulink-PS Converter  PhysicalDomain=network_engine_domain  SubClassName=ps_input  LeftPortType=input  RightPortType=output  PseudoPeriodic=off  Frequencies=[]  NoiseDistribution=none  NoiseParameters=[]  Unit=1  AffineConversion=off  InputFiltering=off  SimscapeFilterOrder=1  InputFilterTimeConstant=.001  UdotUserProvided=0
  Variable Ratio Transmission : sdl_lib/Couplings & Drives/Variable Ratio Transmission  rotation_direction=2  kp=DCT_Param.Transmission.Abstract.Compliance N*m/rad  kv=DCT_Param.Transmission.Abstract.Damping N*m/(rad/s)  initial_torque=0 N*m  losses_model=1  efficiency=0.85  mu_visc=[ 0 0 ] N*m/(rad/s)  w_thr=0.01 rad/s
  Shaft : PMIOPort  Port=1  Side=Left
  F : PMIOPort  Port=2  Side=Right
  wires:
  [nG] -> Ratio Selection/2(nextGear)
  G/1 -> Bus Selector/1
  Bus Selector/1 -> [A1]  "<U1>"
  Bus Selector/2 -> [A2]  "<U2>"
  Bus Selector/3 -> [A3]  "<U3>"
  Bus Selector/4 -> [A4]  "<U4>"
  Bus Selector/5 -> [A5]  "<U5>"
  Bus Selector/6 -> [A6]  "<U6>"
  Bus Selector/7 -> [AR]  "<UR>"
  Ratio Selection/1(Ratio) -> Simulink-PS Converter/1
  [G] -> Ratio Selection/1(Gear)
  connections:
  Variable Ratio Transmission/LConn2 -- Shaft/RConn1
  Variable Ratio Transmission/RConn1 -- Gear Inertia/LConn1 -- F/RConn1
  Simulink-PS Converter/RConn1 -- Variable Ratio Transmission/LConn1

== system Dual_Clutch_Trans_SDO_ORIG/Engine/Torque Sensor ==
  Ideal Torque Sensor : fl_lib/Mechanical/Mechanical Sensors/Ideal Torque Sensor
  PS-Simulink Converter1 : nesl_utility/PS-Simulink Converter  PhysicalDomain=network_engine_domain  SubClassName=ps_output  LeftPortType=input  RightPortType=output  PseudoPeriodic=off  Frequencies=[]  Unit=N*m  AffineConversion=off
  R : PMIOPort  Port=1  Side=Left
  C : PMIOPort  Port=2  Side=Right
  tag scope: EngTrq_Nm=global
  wires:
  PS-Simulink Converter1/1 -> [EngTrq_Nm]
  connections:
  R/RConn1 -- Ideal Torque Sensor/LConn1
  C/RConn1 -- Ideal Torque Sensor/RConn1
  Ideal Torque Sensor/RConn2 -- PS-Simulink Converter1/LConn1

== system Dual_Clutch_Trans_SDO_ORIG/Engine/Velocity sensor ==
  Ideal Rotational Motion Sensor : fl_lib/Mechanical/Mechanical Sensors/Ideal Rotational Motion Sensor  offset=0 rad
  MRR : fl_lib/Mechanical/Rotational Elements/Mechanical Rotational Reference
  PS2S : nesl_utility/PS-Simulink Converter  PhysicalDomain=network_engine_domain  SubClassName=ps_output  LeftPortType=input  RightPortType=output  PseudoPeriodic=off  Frequencies=[]  Unit=rpm  AffineConversion=off
  Sensor dynamics : TransferFcn  Denominator=[0.01 1]
  Zero-Order Hold : ZeroOrderHold  SampleTime=0.01
  F : PMIOPort  Port=1  Side=Left
  rpm : Outport
  wires:
  PS2S/1 -> Sensor dynamics/1
  Sensor dynamics/1 -> Zero-Order Hold/1
  Zero-Order Hold/1 -> rpm/1
  connections:
  F/RConn1 -- Ideal Rotational Motion Sensor/LConn1
  Ideal Rotational Motion Sensor/RConn2 -- PS2S/LConn1
  MRR/LConn1 -- Ideal Rotational Motion Sensor/RConn1

== system Dual_Clutch_Trans_SDO_ORIG/Engine Management/Inverse engine map ==
  EngSpd : Inport
  trq_demand : Inport  Port=2
  Product : Product  SaturateOnIntegerOverflow=on  InputSameDT=on  OutDataTypeStr=Inherit: Same as first input
  Product1 : Product  Inputs=3  SaturateOnIntegerOverflow=on  InputSameDT=on  OutDataTypeStr=Inherit: Same as first input
  Product2 : Product  Inputs=*/  SaturateOnIntegerOverflow=on  InputSameDT=on  OutDataTypeStr=Inherit: Same as first input
  Sum1 : Sum  Inputs=|++  SaturateOnIntegerOverflow=on  InputSameDT=on  OutDataTypeStr=Inherit: Same as first input
  Sum2 : Sum  Inputs=|+-  SaturateOnIntegerOverflow=on  InputSameDT=on  OutDataTypeStr=Inherit: Same as first input
  p1 : Constant  Value=P0/w0
  p2 : Constant  Value=P0/w0^2
  p3 : Constant  Value=P0/w0^3
  rpm2rad/s : Gain  Gain=2*pi/60  SaturateOnIntegerOverflow=on  OutDataTypeStr=Inherit: Same as input  ParamDataTypeStr=Inherit: Same as input
  throttle : Outport
  wires:
  p1/1 -> Sum1/1
  Sum2/1 -> Product2/2  "Tmax"
  Product2/1 -> throttle/1
  Product1/1 -> Sum2/2
  Sum1/1 -> Sum2/1
  p3/1 -> Product1/3
  Product/1 -> Sum1/2
  p2/1 -> Product/2
  rpm2rad/s/1 -> Product1/2, Product1/1, Product/1
  trq_demand/1 -> Product2/1
  EngSpd/1 -> rpm2rad/s/1

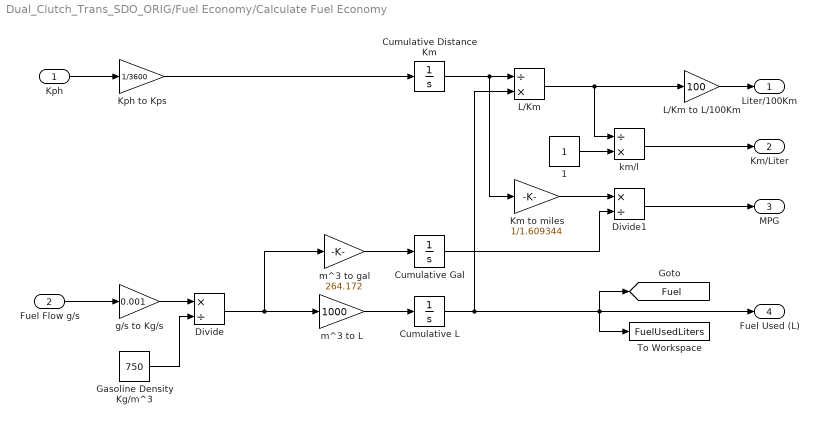
== system Dual_Clutch_Trans_SDO_ORIG/Fuel Economy/Calculate Fuel Economy ==
  Kph : Inport
  Fuel Flow g/s : Inport  Port=2
  1 : Constant
  Cumulative Distance Km : Integrator  InitialCondition=eps
  Cumulative Gal : Integrator  InitialCondition=eps
  Cumulative L : Integrator  InitialCondition=eps
  Divide : Product  Inputs=*/
  Divide1 : Product  Inputs=*/
  Gasoline Density Kg/m^3 : Constant  Value=750
  Km to miles : Gain  Gain=1/1.609344
  Kph to Kps : Gain  Gain=1/3600
  L/Km : Product  Inputs=/*
  L/Km to L/100Km : Gain  Gain=100
  To Workspace : ToWorkspace  VariableName=FuelUsedLiters  SampleTime=-1
      settings: MaxDataPoints=1
  g/s to Kg/s : Gain  Gain=0.001
  km/l : Product  Inputs=/*
  m^3 to L : Gain  Gain=1000
  m^3 to gal : Gain  Gain=264.172
  Liter/100Km : Outport
  Km/Liter : Outport  Port=2
  MPG : Outport  Port=3
  Fuel Used (L) : Outport  Port=4
  tag scope: Fuel=global
  wires:
  km/l/1 -> Km/Liter/1
  1/1 -> km/l/2
  Divide1/1 -> MPG/1
  L/Km to L/100Km/1 -> Liter/100Km/1
  Fuel Flow g/s/1 -> g/s to Kg/s/1
  Kph/1 -> Kph to Kps/1
  Cumulative Gal/1 -> Divide1/2
  Km to miles/1 -> Divide1/1
  L/Km/1 -> km/l/1, L/Km to L/100Km/1
  Cumulative Distance Km/1 -> Km to miles/1, L/Km/1
  Cumulative L/1 -> L/Km/2, Fuel Used (L)/1, To Workspace/1, [Fuel]
  Kph to Kps/1 -> Cumulative Distance Km/1
  m^3 to gal/1 -> Cumulative Gal/1
  m^3 to L/1 -> Cumulative L/1
  Divide/1 -> m^3 to gal/1, m^3 to L/1
  Gasoline Density Kg/m^3/1 -> Divide/2
  g/s to Kg/s/1 -> Divide/1

== system Dual_Clutch_Trans_SDO_ORIG/Speed Demand/10-15 mode  ==
  Demux : Demux  Tag=STV Demux  Outputs=1
  FromWs : FromWorkspace  Tag=STV FromWs  VariableName=tuvar  SampleTime=0
      SigBuilderData=|
      | common.afterFinalStr = 'Extrapolate'
      | common.sampleTime = '0'
      | dataSet.timeRange = [0 660]
      | dataSet.name = '10-15 Mode Cycle'
      | sbobj.Groups.Name = '10-15 Mode Cycle'
      | sbobj.Groups.Signals.Name = 'Target speed'
      | sbobj.Groups.Signals.XData = [0 44 51 66 73 89 103 118 128 130 142 152 159 179 186 201 208 224 238 253 263 265 277 287 294 314 321 336 343 359 373 388 398 400 412 422 429 494 512 524 528 532 548 558 569 579 589 593 615 620 640 650 660]
      | sbobj.Groups.Signals.YData = [0 0 20 20 0 0 40 40 20 20 40 20 0 0 20 20 0 0 40 40 20 20 40 20 0 0 20 20 0 0 40 40 20 20 40 20 0 0 50 50 40 40 60 60 70 70 50 50 70 70 30 0 0]
  Target speed : Outport  Tag=STV Outport
  wires:
  Demux/1 -> Target speed/1
  FromWs/1 -> Demux/1

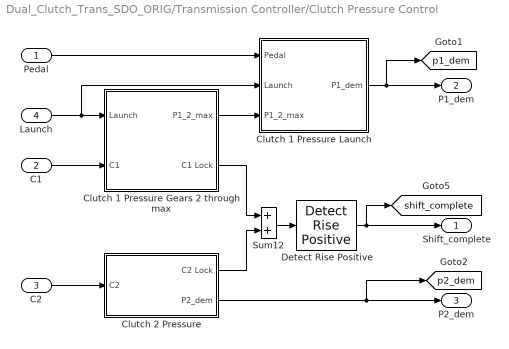
== system Dual_Clutch_Trans_SDO_ORIG/Transmission Controller/Clutch Pressure Control ==
  Pedal : Inport
  C1 : Inport  Port=2
  C2 : Inport  Port=3
  Launch : Inport  Port=4
  Clutch 1 Pressure Gears 2 through max : Subsystem
  Clutch 1 Pressure Launch : Subsystem
  Clutch 2 Pressure : Subsystem
  Detect Rise Positive : simulink/Logic and Bit Operations/Detect Rise Positive  vinit=0  InputProcessing=Inherited  OutDataTypeStr=uint8
  Sum12 : Sum  SaturateOnIntegerOverflow=on  InputSameDT=on  OutDataTypeStr=Inherit: Same as first input
  Shift_complete : Outport  OutputWhenDisabled=reset  InitialOutput=0
  P1_dem : Outport  Port=2  OutputWhenDisabled=reset  InitialOutput=0
  P2_dem : Outport  Port=3  OutputWhenDisabled=reset  InitialOutput=0
  tag scope: p1_dem=global, p2_dem=global, shift_complete=global
  wires:
  C2/1 -> Clutch 2 Pressure/1(C2)
  Clutch 2 Pressure/2(P2_dem) -> [p2_dem], P2_dem/1
  Clutch 1 Pressure Launch/1(P1_dem) -> P1_dem/1, [p1_dem]
  Sum12/1 -> Detect Rise Positive/1
  Detect Rise Positive/1 -> Shift_complete/1, [shift_complete]
  Clutch 1 Pressure Gears 2 through max/1(P1_2_max) -> Clutch 1 Pressure Launch/3(P1_2_max)
  C1/1 -> Clutch 1 Pressure Gears 2 through max/2(C1)
  Launch/1 -> Clutch 1 Pressure Gears 2 through max/1(Launch), Clutch 1 Pressure Launch/2(Launch)
  Clutch 1 Pressure Gears 2 through max/2(C1 Lock) -> Sum12/1
  Pedal/1 -> Clutch 1 Pressure Launch/1(Pedal)
  Clutch 2 Pressure/1(C2 Lock) -> Sum12/2

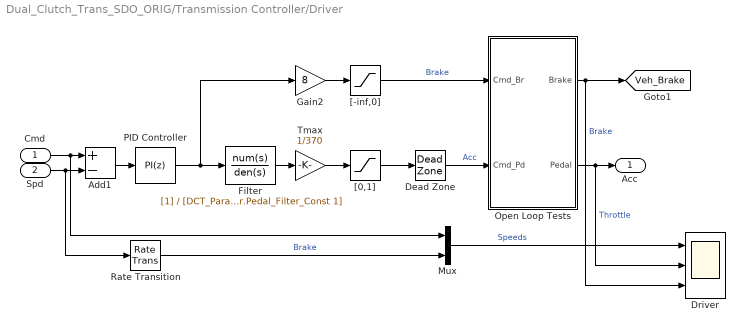
== system Dual_Clutch_Trans_SDO_ORIG/Transmission Controller/Driver ==
  Cmd : Inport
  Spd : Inport  Port=2
  Add1 : Sum  Inputs=+-  SampleTime=0.01
  Dead Zone : DeadZone  LowerValue=0  UpperValue=2e-2  SaturateOnIntegerOverflow=on
  Driver : Scope  NumInputPorts=3
  Filter : TransferFcn  Denominator=[DCT_Param.Driver.Pedal_Filter_Const 1]
  Gain2 : Gain  Gain=8
  Mux : Mux  Inputs=2
  Open Loop Tests : Subsystem
  PID Controller : simulink/Continuous/PID Controller  Controller=PI  TimeDomain=Discrete-time  SampleTime=-1  IntegratorMethod=Forward Euler  FilterMethod=Forward Euler  Form=Parallel  UseFilter=on  ControllerParametersSource=internal  P=DCT_Param.Driver.Kp  I=DCT_Param.Driver.Ki  D=0  N=100  InitialConditionSource=internal  InitialConditionForIntegrator=0  InitialConditionForFilter=0  ExternalReset=none  LimitOutput=off  UpperSaturationLimit=inf  LowerSaturationLimit=-inf  LinearizeAsGain=off  AntiWindupMode=none  Kb=1  TrackingMode=off  Kt=1  PParamMin=[]  PParamMax=[]  IParamMin=[]  IParamMax=[]  DParamMin=[]  DParamMax=[]  NParamMin=[]  NParamMax=[]  KbParamMin=[]  KbParamMax=[]  KtParamMin=[]  KtParamMax=[]  POutMin=[]  POutMax=[]  IOutMin=[]  IOutMax=[]  DOutMin=[]  DOutMax=[]  NOutMin=[]  NOutMax=[]  KbOutMin=[]  KbOutMax=[]  KtOutMin=[]  KtOutMax=[]  IntegratorOutMin=[]  IntegratorOutMax=[]  FilterOutMin=[]  FilterOutMax=[]  SumOutMin=[]  SumOutMax=[]  SumI1OutMin=[]  SumI1OutMax=[]  SumI2OutMin=[]  SumI2OutMax=[]  SumI3OutMin=[]  SumI3OutMax=[]  SumDOutMin=[]  SumDOutMax=[]  SaturationOutMin=[]  SaturationOutMax=[]  IntegratorContinuousStateAttributes=''  IntegratorStateMustResolveToSignalObject=off  IntegratorRTWStateStorageClass=Auto  FilterContinuousStateAttributes=''  FilterStateMustResolveToSignalObject=off  FilterRTWStateStorageClass=Auto  DifferentiatorICPrevScaledInput=0  DifferentiatorOutMin=[]  DifferentiatorOutMax=[]
  Rate Transition : RateTransition
  Tmax : Gain  Gain=1/370  SaturateOnIntegerOverflow=on  OutDataTypeStr=Inherit: Same as input  ParamDataTypeStr=Inherit: Same as input
  "[-inf,0]" : Saturate  UpperLimit=0  LowerLimit=-inf
  "[0,1]" : Saturate  UpperLimit=1  LowerLimit=0
  Acc : Outport
  tag scope: Veh_Brake=global
  wires:
  "[0,1]"/1 -> Dead Zone/1
  Cmd/1 -> Mux/1, Add1/1
  Spd/1 -> Add1/2, Rate Transition/1
  "[-inf,0]"/1 -> Open Loop Tests/1(Cmd_Br)  "Brake"
  Add1/1 -> PID Controller/1
  Tmax/1 -> "[0,1]"/1
  PID Controller/1 -> Filter/1, Gain2/1
  Open Loop Tests/1(Brake) -> Driver/3, [Veh_Brake]  "Brake"
  Mux/1 -> Driver/1  "Speeds"
  Gain2/1 -> "[-inf,0]"/1
  Dead Zone/1 -> Open Loop Tests/2(Cmd_Pd)  "Acc"
  Open Loop Tests/2(Pedal) -> Driver/2, Acc/1  "Throttle"
  Rate Transition/1 -> Mux/2  "Brake"
  Filter/1 -> Tmax/1

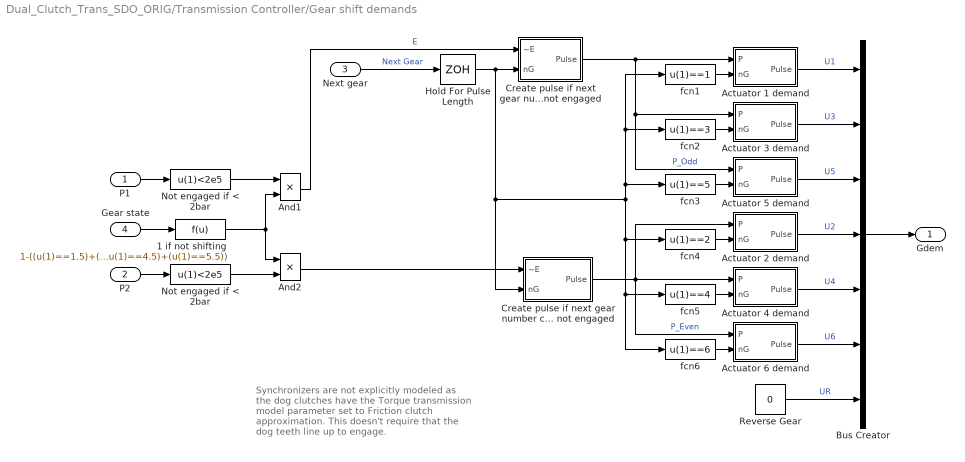
== system Dual_Clutch_Trans_SDO_ORIG/Transmission Controller/Gear shift demands ==
  note: Synchronizers are not explicitly
      | modeled as the dog clutches have
      | the Torque transmission model
      | parameter set to Friction clutch
      | approximation. This doesn't require
      | that the dog teeth line up to
      | engage.
  P1 : Inport
  P2 : Inport  Port=2
  Next gear : Inport  Port=3
  Gear state : Inport  Port=4
  1 if not shifting : Fcn  Expr=1-((u(1)==1.5)+(u(1)==2.5)+(u(1)==3.5)+(u(1)==4.5)+(u(1)==5.5))
  Actuator 1 demand : Subsystem
  Actuator 2 demand : Subsystem
  Actuator 3 demand : Subsystem
  Actuator 4 demand : Subsystem
  Actuator 5 demand : Subsystem
  Actuator 6 demand : Subsystem
  And1 : Product  SaturateOnIntegerOverflow=on  InputSameDT=on  OutDataTypeStr=Inherit: Same as first input
  And2 : Product  SaturateOnIntegerOverflow=on  InputSameDT=on  OutDataTypeStr=Inherit: Same as first input
  Bus Creator : BusCreator  Inputs=7
  Create pulse if next gear number changes and CL1 is not engaged : Subsystem
  Create pulse if next gear number changes and CL2 is not engaged : Subsystem
  Hold For Pulse Length : ZeroOrderHold  SampleTime=DCT_Param.Dog_Clutches.Pulse_Length*0.01
  Not engaged if < 2bar : Fcn  Expr=u(1)<2e5
  "Not engaged if < 2bar " : Fcn  Expr=u(1)<2e5
  Reverse Gear : Constant  Value=0  SampleTime=0.01
  fcn1 : Fcn  Expr=u(1)==1
  fcn2 : Fcn  Expr=u(1)==3
  fcn3 : Fcn  Expr=u(1)==5
  fcn4 : Fcn  Expr=u(1)==2
  fcn5 : Fcn  Expr=u(1)==4
  fcn6 : Fcn  Expr=u(1)==6
  Gdem : Outport
  wires:
  And2/1 -> Create pulse if next gear number changes and CL2 is not engaged/1(~E)
  And1/1 -> Create pulse if next gear number changes and CL1 is not engaged/1(~E)  "E"
  "Not engaged if < 2bar "/1 -> And2/2
  1 if not shifting/1 -> And2/1, And1/2
  Not engaged if < 2bar/1 -> And1/1
  P2/1 -> "Not engaged if < 2bar "/1
  P1/1 -> Not engaged if < 2bar/1
  Gear state/1 -> 1 if not shifting/1
  Actuator 4 demand/1(Pulse) -> Bus Creator/5  "U4"
  Actuator 2 demand/1(Pulse) -> Bus Creator/4  "U2"
  Create pulse if next gear number changes and CL2 is not engaged/1(Pulse) -> Actuator 4 demand/1(P), Actuator 2 demand/1(P), Actuator 6 demand/1(P)  "P_Even"
  fcn5/1 -> Actuator 4 demand/2(nG)
  fcn4/1 -> Actuator 2 demand/2(nG)
  Actuator 5 demand/1(Pulse) -> Bus Creator/3  "U5"
  Actuator 3 demand/1(Pulse) -> Bus Creator/2  "U3"
  Create pulse if next gear number changes and CL1 is not engaged/1(Pulse) -> Actuator 5 demand/1(P), Actuator 3 demand/1(P), Actuator 1 demand/1(P)  "P_Odd"
  fcn3/1 -> Actuator 5 demand/2(nG)
  fcn2/1 -> Actuator 3 demand/2(nG)
  fcn1/1 -> Actuator 1 demand/2(nG)
  Next gear/1 -> Hold For Pulse Length/1  "Next Gear"
  Actuator 1 demand/1(Pulse) -> Bus Creator/1  "U1"
  Bus Creator/1 -> Gdem/1
  fcn6/1 -> Actuator 6 demand/2(nG)
  Actuator 6 demand/1(Pulse) -> Bus Creator/6  "U6"
  Reverse Gear/1 -> Bus Creator/7  "UR"
  Hold For Pulse Length/1 -> Create pulse if next gear number changes and CL1 is not engaged/2(nG), Create pulse if next gear number changes and CL2 is not engaged/2(nG), fcn4/1, fcn5/1, fcn6/1, fcn3/1, fcn2/1, fcn1/1
